simulink model "blocks"  (R2018b)
settings: Solver=ode45  StartTime=0.0  StopTime=10.0  RelTol=1e-3  AbsTol=1e-6
undefined symbols (not defined in the file): C, L, R
settings Model: ExtModeTrigMode=oneshot  ExtModeArmWhenConnect=off  Creator=eechris  LastModifiedBy=eechris
settings DataIOCC: SaveFormat=Array  SignalLoggingSaveFormat=ModelDataLogs
settings OptimizationCC: BlockReduction=off  BooleanDataType=off
settings DebuggingCC: SaveWithParameterizedLinksMsg=none  UnderspecifiedInitializationDetection=Classic  MergeDetectMultiDrivingBlocksExec=none  SignalResolutionControl=TryResolveAllWithWarning  MultiTaskDSMMsg=warning  MultiTaskCondExecSysMsg=none
settings HardwareCC: TargetUnknown=on
settings ModelReferenceCC: PropagateSignalLabelsOutOfModel=off
settings GRTTargetCC: CombineOutputUpdateFcns=off  GRTInterface=on

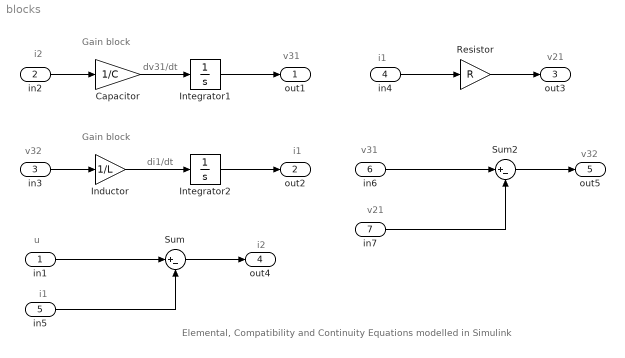
== system blocks ==
  note: dv31/dt
  note: v31
  note: Gain block
  note: di1/dt
  note: i1
  note: Gain block
  note: i2
  note: i1
  note: v21
  note: v32
  note: u
  note: i1
  note: i2
  note: v31
  note: v21
  note: v32
  note: Elemental, Compatibility and Continuity Equations modelled in Simulink
  in1 : Inport
  in2 : Inport  Port=2
  in3 : Inport  Port=3
  in4 : Inport  Port=4
  in5 : Inport  Port=5
  in6 : Inport  Port=6
  in7 : Inport  Port=7
  Capacitor : Gain  Gain=1/C  OutDataTypeStr=Inherit: Same as input  ParamDataTypeStr=Inherit: Same as input
  Inductor : Gain  Gain=1/L  OutDataTypeStr=Inherit: Same as input  ParamDataTypeStr=Inherit: Same as input
  Integrator1 : Integrator
  Integrator2 : Integrator
  Resistor : Gain  Gain=R  SaturateOnIntegerOverflow=on  OutDataTypeStr=Inherit: Same as input  ParamDataTypeStr=Inherit: Same as input
  Sum : Sum  Inputs=|+-  InputSameDT=on  OutDataTypeStr=Inherit: Same as first input
  Sum2 : Sum  Inputs=|+-  InputSameDT=on  OutDataTypeStr=Inherit: Same as first input
  out1 : Outport
  out2 : Outport  Port=2
  out3 : Outport  Port=3
  out4 : Outport  Port=4
  out5 : Outport  Port=5
  wires:
  Capacitor/1 -> Integrator1/1
  in2/1 -> Capacitor/1
  Integrator1/1 -> out1/1
  Inductor/1 -> Integrator2/1
  in3/1 -> Inductor/1
  Integrator2/1 -> out2/1
  in4/1 -> Resistor/1
  Resistor/1 -> out3/1
  in6/1 -> Sum2/1
  Sum2/1 -> out5/1
  in7/1 -> Sum2/2
  in1/1 -> Sum/1
  Sum/1 -> out4/1
  in5/1 -> Sum/2
